simulink model "MotorControlTest"  (R2017b)
settings: Solver=VariableStepAuto  StartTime=0.0  StopTime=5  RelTol=1e-3
libraries: simulink x1
settings Model: Creator=hoang  LastModifiedBy=hoang

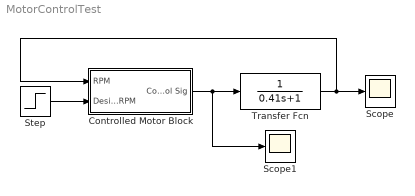
== system MotorControlTest ==
  Controlled Motor Block : Subsystem  mask{k=0.45, Km=1, Ts=0.02, T=0.41, Rdt=6.22, Rdx=1}
      mask prompts: k "Velocity Gain (k)"; Km "Motor Amplification (Km)"; Ts "Sampling Time (Ts)"; T "Motor Time Constant (T)"; Rdt "Maximum Output Threshold (Rdt)"; Rdx "Maximum Derivative Threshold (Rdx)"
      settings: OpenFcn=set_param(gcbh,'LinkStatus','none');
  Scope : Scope
  Scope1 : Scope
  Step : Step  SampleTime=0
  Transfer Fcn : TransferFcn  Denominator=[0.41 1]
  wires:
  Step/1 -> Controlled Motor Block/2(DesiredRPM)
  Controlled Motor Block/1(Control Sig) -> Scope1/1, Transfer Fcn/1
  Transfer Fcn/1 -> Controlled Motor Block/1(RPM), Scope/1

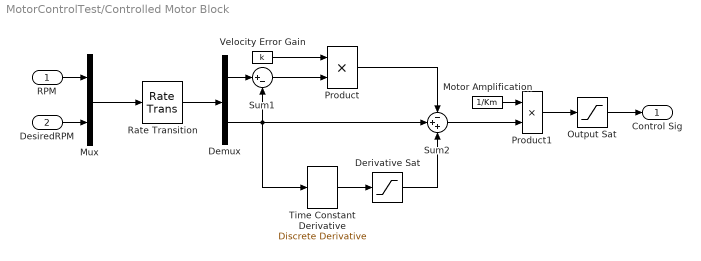
== system MotorControlTest/Controlled Motor Block ==
  RPM : Inport
  DesiredRPM : Inport  Port=2
  Demux : Demux  Outputs=2
  Derivative Sat : Saturate  UpperLimit=Rdx  LowerLimit=-Rdx
  Motor Amplification : Constant  Value=1/Km
  Mux : Mux  Inputs=2
  Output Sat : Saturate  UpperLimit=Rdt  LowerLimit=0
  Product : Product
  Product1 : Product
  Rate Transition : RateTransition  OutPortSampleTime=Ts
  Sum1 : Sum  Inputs=|+-
  Sum2 : Sum  Inputs=-++
  Time Constant Derivative : simulink/Discrete/Discrete Derivative  gainval=T  ICPrevScaledInput=0.0  OutMin=[]  OutMax=[]  OutDataType=fixdt(1, 16)  OutScaling=2^-10  DoSatur=off
  Velocity Error Gain : Constant  Value=k
  Control Sig : Outport
  wires:
  Derivative Sat/1 -> Sum2/3
  Output Sat/1 -> Control Sig/1
  Time Constant Derivative/1 -> Derivative Sat/1
  Product1/1 -> Output Sat/1
  Motor Amplification/1 -> Product1/1
  Sum2/1 -> Product1/2
  Product/1 -> Sum2/1
  Velocity Error Gain/1 -> Product/1
  Sum1/1 -> Product/2
  Demux/1 -> Sum1/1
  Demux/2 -> Sum1/2, Sum2/2, Time Constant Derivative/1
  Rate Transition/1 -> Demux/1
  Mux/1 -> Rate Transition/1
  DesiredRPM/1 -> Mux/2
  RPM/1 -> Mux/1
